simulink model "MPC"  (R2024b)
settings: Solver=ode4  StartTime=0.0  StopTime=tsim  FixedStep=baseRate  RelTol=1e-6  AbsTol=1e-6
values from neighbouring files (symbols this model uses):
  C = [cos(theta), -sin(theta) ... (first row only)    [Run_Initializer.m]    (also in plotBatch.m = quat2Rotm(q','scalarFirst'))
  camera_FOV = 40*d2r    (= 0.698131700798)    [Run_Initializer.m]
  camera_offset = [0.145, 0.087]'    [Run_Initializer.m]
  docking_face = [0 1]'    [Run_Initializer.m]
  docking_offset = [0 0 0]'    [Run_Initializer.m]
  eta = 0.7    [Run_Initializer.m]
  F_t = [kron(eye(N_h),  [zeros(2,3), eye(2), zeros(2,4)]) ... (first row only)    [Run_Initializer.m]
  f_t = [kron(ones(N_h, 1), [xLength yLength]' - edge_buffer) ... (first row only)    [Run_Initializer.m]
  F_u = [kron(eye(N_h),  [eye(3), zeros(3,6)]) ... (first row only)    [Run_Initializer.m]
  f_u = kron(ones(2*N_h, 1), u_max')    [Run_Initializer.m]
  F_v = [kron(eye(N_h),  [zeros(1,5), 1, zeros(1,3)]) ... (first row only)    [Run_Initializer.m]
  gamma = 0.95    [Run_Initializer.m]
  Gamma1_el = 0.12    [Run_Initializer.m]
  Gamma1_sh = 0.005    [Run_Initializer.m]
  Gamma1_wr = 0.025    [Run_Initializer.m]
  Gamma2_el = 5    [Run_Initializer.m]
  Gamma2_sh = 5    [Run_Initializer.m]
  Gamma2_wr = 5    [Run_Initializer.m]
  Gamma3_el = 10    [Run_Initializer.m]
  Gamma3_sh = 40    [Run_Initializer.m]
  Gamma3_wr = 40    [Run_Initializer.m]
  Gamma4_el = 0.039    [Run_Initializer.m]
  Gamma4_sh = 0.015    [Run_Initializer.m]
  Gamma4_wr = 0.029    [Run_Initializer.m]
  Gamma5_el = 800    [Run_Initializer.m]
  Gamma5_sh = 800    [Run_Initializer.m]
  Gamma5_wr = 800    [Run_Initializer.m]
  Gamma6_el = 0.000001    (= 1e-06)    [Run_Initializer.m]
  Gamma6_sh = 0.005    [Run_Initializer.m]
  Gamma6_wr = 0.02    [Run_Initializer.m]
  H = kron(eye(N_h), [R, zeros(3,6); zeros(6,3), Q])    [Run_Initializer.m]
  IBLACK = 0.1996    [unpackData.m]
  IRED = 0.1982    [unpackData.m]
  J = sum(wp*posErr + wt*angErr)    [find_transformation.m]
  Kd_elarm = 0.8    [Run_Initializer.m]
  Kd_sharm = 1.0    (= 1)    [Run_Initializer.m]
  Kd_wrarm = 0.6    [Run_Initializer.m]
  Kp_elarm = 1.2    [Run_Initializer.m]
  Kp_sharm = 1.5    [Run_Initializer.m]
  Kp_wrarm = 1.0    (= 1)    [Run_Initializer.m]
  m = m + 5    (= 4)    [unpackData.m]
  M = diag([1/m; 1/m; 1/I])    [unpackData.m]
  maxd = [d1 ... (first row only)    [Run_Initializer.m]
  mBLACK = 11.3620    (= 11.362)    [unpackData.m]
  mRED = 11.2970    (= 11.297)    [unpackData.m]
  N = size(rel,1)    [plotBatch.m]    (also in unpackData.m = 0)
  p = [0 obj.pos(k,:)]    [SparseState6DOF.m]
  PDQ = blkdiag(20*eye(3),eye(3), 20*eye(3),eye(3))    [Run_Initializer.m]
  PQ = blkdiag(20*eye(6),eye(6))    [Run_Initializer.m]
  PR = blkdiag(20*eye(3), eye(6), 0.0001*eye(3))    [Run_Initializer.m]
  PWMFreq = 5    [Run_Initializer.m]
  Q = diag([100 100 100 300 300 300])    [Run_Initializer.m]    (also in unpackData.m = blkdiag(0.0001*eye(2), 0.00001))
  R = diag([200 200 200])    [Run_Initializer.m]    (also in plotBatch.m = C3(yaw); unpackData.m = diag([6;6;6]))
  r_hold_obs = 1.1*sqrt(2)*0.3.*[1 1]    [Run_Initializer.m]
  r_hold_tar_min = [0.8; (0.3+0.05)]    [Run_Initializer.m]
  rho = 0.98    [Run_Initializer.m]
  T_d = 2    [Run_Initializer.m]
  T_max = 0.15    [Run_Initializer.m]
  Tz_lim_elarm = .1    (= 0.1)    [Run_Initializer.m]
  Tz_lim_sharm = .1    (= 0.1)    [Run_Initializer.m]
  Tz_lim_wrarm = .1    (= 0.1)    [Run_Initializer.m]
  use_LOS_constr = 1    [Run_Initializer.m]
  use_table_constr = 1    [Run_Initializer.m]
  x_BLACK_0 = [(1/3)*xLength (1/3)*yLength-0.2 280*d2r 0.01 0.005 1.88*d2r]'    [Run_Initializer.m]
  x_BLUE_0 = [0 0 0 0 0 0]'    [Run_Initializer.m]
  zeta = 10*d2r    (= 0.174532925199)    [Run_Initializer.m]
undefined symbols (not defined in the file or in its folder): a1, a2, a3, alpha, alpha_m, alpha_t, alphas, alphas_t, alphat, Am, b, b0, b1, b2, b3, baseRate, Bm, c, c1, c1t, c2, c2t, Cm, d, dataRate, DiscIntNeverNeededParam, Dm, drop_states_ARM, drop_states_BLACK, drop_states_BLUE, drop_states_RED, epsilon, epsilont, F_black_X_nominal, F_black_Y_nominal, F_blue_X_nominal, F_blue_Y_nominal, F_max, F_red_X_nominal, F_red_Y_nominal, F_thrusters_BLACK, F_thrusters_BLUE, F_thrusters_RED, gamma_I, gamma_I_t, gamma_P, gamma_P_t, home_states_BLACK, home_states_BLUE, home_states_RED, IBLUE, IDIST, IEE, init_states_BLACK, init_states_BLUE, init_states_RED, IPROX, k, K, k1 ... (+62)
libraries: simulink x33, nvidiaSharedBlocks x13, slpidlib x6, MainLibrary x5, dspsigops x3, dspinverses x3, nvidiaIMUSensorslib x1
(part 10 of 12)

== system MPC/Thruster Control Code/Change RED Behavior/Calculate Duty Cycle/Duty Cycle @ PWM/Enabled Subsystem1 ==
  ThrustPer_Final : Inport
  Enable : EnablePort
  Out1 : Outport
  wires:
  ThrustPer_Final/1 -> Out1/1

== system MPC/1 - Experiment Logic/Phase #3: Experiment/Sub-Phase #1/Desired Position BLACK/Calculate Time since Phase #3 Start/Subsystem ==
  Universal_Time : DataStoreRead  DataStoreName=Univ_Time  IndexOptions=Index vector (dialog)  Indices=1  OutputSizes=1
  Time : Outport  VectorParamsAs1DForOutWhenUnconnected=off
  wires:
  Universal_Time/1 -> Time/1

== system MPC/1 - Experiment Logic/Phase #3: Experiment/Sub-Phase #1/Desired Position BLUE/Calculate Time since Phase #3 Start/Subsystem ==
  Universal_Time : DataStoreRead  DataStoreName=Univ_Time  IndexOptions=Index vector (dialog)  Indices=1  OutputSizes=1
  Time : Outport  VectorParamsAs1DForOutWhenUnconnected=off
  wires:
  Universal_Time/1 -> Time/1

== system MPC/1 - Experiment Logic/Phase #3: Experiment/Sub-Phase #3 /Desired Position BLACK/Calculate Time since Phase #3 Start/Subsystem ==
  Universal_Time : DataStoreRead  DataStoreName=Univ_Time  IndexOptions=Index vector (dialog)  Indices=1  OutputSizes=1
  Time : Outport  VectorParamsAs1DForOutWhenUnconnected=off
  wires:
  Universal_Time/1 -> Time/1

== system MPC/1 - Experiment Logic/Phase #3: Experiment/Sub-Phase #4/Desired Position BLACK/Calculate Time since Phase #3 Start/Subsystem ==
  Universal_Time : DataStoreRead  DataStoreName=Univ_Time  IndexOptions=Index vector (dialog)  Indices=1  OutputSizes=1
  Time : Outport  VectorParamsAs1DForOutWhenUnconnected=off
  wires:
  Universal_Time/1 -> Time/1

== system MPC/4 - Control/Default PD Control (RED)/SAC/SAC_CTL/Position/Storage ==
  u : Inport
  In2 : Inport  Port=2
  u1 : Inport  Port=3
  Data Store Write : DataStoreWrite  DataStoreName=SAC_ke_1  IndexOptions=Index vector (dialog)  Indices=1  OutputSizes=1
  Data Store Write1 : DataStoreWrite  DataStoreName=SAC_kx_1  IndexOptions=Index vector (dialog)  Indices=1  OutputSizes=1
  Data Store Write10 : DataStoreWrite  DataStoreName=SAC_kx_3  IndexOptions=Index vector (dialog)  Indices=1  OutputSizes=1
  Data Store Write11 : DataStoreWrite  DataStoreName=SAC_kx_4  IndexOptions=Index vector (dialog)  Indices=1  OutputSizes=1
  Data Store Write12 : DataStoreWrite  DataStoreName=SAC_kx_5  IndexOptions=Index vector (dialog)  Indices=1  OutputSizes=1
  Data Store Write13 : DataStoreWrite  DataStoreName=SAC_kx_6  IndexOptions=Index vector (dialog)  Indices=1  OutputSizes=1
  Data Store Write14 : DataStoreWrite  DataStoreName=SAC_kx_7  IndexOptions=Index vector (dialog)  Indices=1  OutputSizes=1
  Data Store Write15 : DataStoreWrite  DataStoreName=SAC_kx_8  IndexOptions=Index vector (dialog)  Indices=1  OutputSizes=1
  Data Store Write2 : DataStoreWrite  DataStoreName=SAC_ku_1  IndexOptions=Index vector (dialog)  Indices=1  OutputSizes=1
  Data Store Write3 : DataStoreWrite  DataStoreName=SAC_ke_2  IndexOptions=Index vector (dialog)  Indices=1  OutputSizes=1
  Data Store Write4 : DataStoreWrite  DataStoreName=SAC_ke_3  IndexOptions=Index vector (dialog)  Indices=1  OutputSizes=1
  Data Store Write5 : DataStoreWrite  DataStoreName=SAC_ke_4  IndexOptions=Index vector (dialog)  Indices=1  OutputSizes=1
  Data Store Write6 : DataStoreWrite  DataStoreName=SAC_ku_2  IndexOptions=Index vector (dialog)  Indices=1  OutputSizes=1
  Data Store Write7 : DataStoreWrite  DataStoreName=SAC_ku_3  IndexOptions=Index vector (dialog)  Indices=1  OutputSizes=1
  Data Store Write8 : DataStoreWrite  DataStoreName=SAC_ku_4  IndexOptions=Index vector (dialog)  Indices=1  OutputSizes=1
  Data Store Write9 : DataStoreWrite  DataStoreName=SAC_kx_2  IndexOptions=Index vector (dialog)  Indices=1  OutputSizes=1
  MATLAB Function : MATLAB Function  TreatAsAtomicUnit=on
  MATLAB Function1 : MATLAB Function  TreatAsAtomicUnit=on
  MATLAB Function2 : MATLAB Function  TreatAsAtomicUnit=on
  MATLAB Function3 : MATLAB Function  TreatAsAtomicUnit=on
  MATLAB Function4 : MATLAB Function  TreatAsAtomicUnit=on
  wires:
  MATLAB Function2/3(y3) -> Data Store Write7/1
  u1/1 -> MATLAB Function2/1(u)
  MATLAB Function/3(y3) -> Data Store Write4/1
  MATLAB Function2/4(y4) -> Data Store Write8/1
  MATLAB Function2/1(y1) -> Data Store Write2/1
  MATLAB Function/4(y4) -> Data Store Write5/1
  MATLAB Function/1(y1) -> Data Store Write/1
  MATLAB Function/2(y2) -> Data Store Write3/1
  MATLAB Function2/2(y2) -> Data Store Write6/1
  u/1 -> MATLAB Function/1(u)
  MATLAB Function3/1(y1) -> Data Store Write1/1
  In2/1 -> MATLAB Function4/1(u)
  MATLAB Function4/1(y1) -> MATLAB Function3/1(u)
  MATLAB Function4/2(y2) -> MATLAB Function1/1(u)
  MATLAB Function3/2(y2) -> Data Store Write9/1
  MATLAB Function3/3(y3) -> Data Store Write10/1
  MATLAB Function1/1(y1) -> Data Store Write12/1
  MATLAB Function3/4(y4) -> Data Store Write11/1
  MATLAB Function1/2(y2) -> Data Store Write13/1
  MATLAB Function1/3(y3) -> Data Store Write14/1
  MATLAB Function1/4(y4) -> Data Store Write15/1

== system MPC/Simulate Plant Dynamics/RED and ARM Dynamics/RED + ARM/Calculated & Store Measured States/Subsystem3/Enabled Subsystem ==
  y : Inport
  dt : Inport  Port=2
  Enable : EnablePort
  Constant2 : Constant  Value=0.1
  Delay : Delay  DelayLength=1  InitialConditionSource=Input port
      settings: InputPortMap=u0,p4
  Delay1 : Delay  DelayLength=1
  MATLAB Function : MATLAB Function  TreatAsAtomicUnit=on
  dy/dt : Outport
  wires:
  Constant2/1 -> MATLAB Function/3(tau)
  dt/1 -> MATLAB Function/2(dt)
  Delay/1 -> MATLAB Function/5(ema_prev)
  Delay1/1 -> MATLAB Function/4(dy_prev)
  MATLAB Function/2(ema) -> Delay/1
  y/1 -> MATLAB Function/1(y), Delay/2
  MATLAB Function/1(dy) -> Delay1/1, dy/dt/1

== system MPC/Simulate Plant Dynamics/RED and ARM Dynamics/RED + ARM/Calculated & Store Measured States/Subsystem4/Enabled Subsystem ==
  y : Inport
  dt : Inport  Port=2
  Enable : EnablePort
  Constant2 : Constant  Value=0.1
  Delay : Delay  DelayLength=1  InitialConditionSource=Input port
      settings: InputPortMap=u0,p4
  Delay1 : Delay  DelayLength=1
  MATLAB Function : MATLAB Function  TreatAsAtomicUnit=on
  dy/dt : Outport
  wires:
  Constant2/1 -> MATLAB Function/3(tau)
  dt/1 -> MATLAB Function/2(dt)
  Delay/1 -> MATLAB Function/5(ema_prev)
  Delay1/1 -> MATLAB Function/4(dy_prev)
  MATLAB Function/2(ema) -> Delay/1
  y/1 -> MATLAB Function/1(y), Delay/2
  MATLAB Function/1(dy) -> Delay1/1, dy/dt/1

== system MPC/Simulate Plant Dynamics/RED and ARM Dynamics/RED + ARM/Calculated & Store Measured States/Subsystem5/Enabled Subsystem ==
  y : Inport
  dt : Inport  Port=2
  Enable : EnablePort
  Constant2 : Constant  Value=0.1
  Delay : Delay  DelayLength=1  InitialConditionSource=Input port
      settings: InputPortMap=u0,p4
  Delay1 : Delay  DelayLength=1
  MATLAB Function : MATLAB Function  TreatAsAtomicUnit=on
  dy/dt : Outport
  wires:
  Constant2/1 -> MATLAB Function/3(tau)
  dt/1 -> MATLAB Function/2(dt)
  Delay/1 -> MATLAB Function/5(ema_prev)
  Delay1/1 -> MATLAB Function/4(dy_prev)
  MATLAB Function/2(ema) -> Delay/1
  y/1 -> MATLAB Function/1(y), Delay/2
  MATLAB Function/1(dy) -> Delay1/1, dy/dt/1

== system MPC/Simulate Plant Dynamics/RED and ARM Dynamics/RED + ARM/Data @ Measurement Rate/Calculate True Time Step/Enabled Subsystem3 ==
  y2-y1 : Inport
  Enable : EnablePort
  dy(t)/dt : Outport
  wires:
  y2-y1/1 -> dy(t)/dt/1

== system MPC/Simulate Plant Dynamics/RED and ARM Dynamics/RED Only/Calculated & Store Measured States/Subsystem1/Enabled Subsystem ==
  y : Inport
  dt : Inport  Port=2
  Enable : EnablePort
  Constant2 : Constant  Value=0.1
  Delay : Delay  DelayLength=1  InitialConditionSource=Input port
      settings: InputPortMap=u0,p4
  Delay1 : Delay  DelayLength=1
  MATLAB Function : MATLAB Function  TreatAsAtomicUnit=on
  dy/dt : Outport
  wires:
  Constant2/1 -> MATLAB Function/3(tau)
  dt/1 -> MATLAB Function/2(dt)
  Delay/1 -> MATLAB Function/5(ema_prev)
  Delay1/1 -> MATLAB Function/4(dy_prev)
  MATLAB Function/2(ema) -> Delay/1
  y/1 -> MATLAB Function/1(y), Delay/2
  MATLAB Function/1(dy) -> Delay1/1, dy/dt/1

== system MPC/Simulate Plant Dynamics/RED and ARM Dynamics/RED Only/Calculated & Store Measured States/Subsystem2/Enabled Subsystem ==
  y : Inport
  dt : Inport  Port=2
  Enable : EnablePort
  Constant2 : Constant  Value=0.1
  Delay : Delay  DelayLength=1  InitialConditionSource=Input port
      settings: InputPortMap=u0,p4
  Delay1 : Delay  DelayLength=1
  MATLAB Function : MATLAB Function  TreatAsAtomicUnit=on
  dy/dt : Outport
  wires:
  Constant2/1 -> MATLAB Function/3(tau)
  dt/1 -> MATLAB Function/2(dt)
  Delay/1 -> MATLAB Function/5(ema_prev)
  Delay1/1 -> MATLAB Function/4(dy_prev)
  MATLAB Function/2(ema) -> Delay/1
  y/1 -> MATLAB Function/1(y), Delay/2
  MATLAB Function/1(dy) -> Delay1/1, dy/dt/1

== system MPC/Simulate Plant Dynamics/RED and ARM Dynamics/RED Only/Data @ Measurement Rate/Calculate True Time Step/Enabled Subsystem3 ==
  y2-y1 : Inport
  Enable : EnablePort
  dy(t)/dt : Outport
  wires:
  y2-y1/1 -> dy(t)/dt/1

== matlab function MPC/Data Logger Subsystem/Subsystem8/MATLAB Function ==
  data: u input; y output
function y = fcn(u)

if anynan(u)
    y = -1*ones(size(u));
else
    y = u;
end
end

== matlab function MPC/3 - Navigation/Subsystem/STQMEKF1/MATLAB Function2 ==
  data: u input; out output
function out = fcn(u)

y = u;

y(1:4) = smallQuat(u(1:4),'scalarFirst');
y(5:7) = -1*u(5:7);

out = [y(1:4); y(8:10); y(5:7); y(11:13)];

== matlab function MPC/3 - Navigation/Subsystem/STRMEKF1/MATLAB Function ==
  data: x input; out output; q input
function out = fcn(x,q)

y = [q;x];
y(1:4) = smallQuat(y(1:4),'scalarFirst');

out = [y(1:7); y(11:13); y(8:10)];

== matlab function MPC/Data Logger Subsystem/Subsystem17/MATLAB Function ==
  data: u input; y output
function y = fcn(u)

if anynan(u)
    y = -1*ones(size(u));
else
    y = u;
end
end

== matlab function MPC/Data Logger Subsystem/Subsystem11/MATLAB Function ==
  data: u input; y output
function y = fcn(u)

if anynan(u)
    y = -1*ones(size(u));
else
    y = u;
end
end

== matlab function MPC/3 - Navigation/Subsystem/STRMEKF1/MATLAB Function1 ==
  data: dt input; RED_yaw input; RED_x input; VIS_R input; VIS_x input; x_est output; Rot_est output; x_prev input; Rot_prev input; P_prev input; P_est output; compT output; y output; NIS output; V_est output; V_prev input; Q parameter; R parameter; maxd parameter
function [x_est, Rot_est, P_est, compT, y, NIS, V_est] = RMEKF(dt, RED_yaw, RED_x, VIS_R, VIS_x, x_prev, Rot_prev, P_prev, V_prev, Q, R, maxd)

s1 = 1e-2; % quat
s2 = 1e-4; % angular vel
s3 = 1e-10; % position
s4 = 1e-7; % velocity
s5 = 0.006; % quat meas 
s6 = 0.001 ; % position meas
s7 = s6; 

d1 = 1.6046;
d2 = 5.5866;
rho = 0.98;

Q = blkdiag(s1*eye(3), s3*eye(3), s4*eye(3), s2*eye(3));


R = blkdiag(s5*eye(3), s6, s7*eye(2));

maxd = 1000*[d1
        d2];

rho = 0.98;

r = 0;
z = VIS_x;
Chaser = [RED_x(1:2); RED_yaw];

tic
[x_est, Rot_est, P_est, y, H, V_est] = runSTRMEKF2(Chaser, z, VIS_R, dt, x_prev, Rot_prev, P_prev, Q, R, V_prev, r, rho, maxd);

compT = toc;

% Calc NIS
Pzz = H*P_est*H' + R;
NIS = y' / Pzz * y;

end

== matlab function MPC/Data Logger Subsystem/Subsystem13/MATLAB Function ==
  data: u input; y output
function y = fcn(u)

if anynan(u)
    y = -1*ones(size(u));
else
    y = u;
end
end

== matlab function MPC/Data Logger Subsystem/Subsystem14/MATLAB Function ==
  data: u input; y output
function y = fcn(u)

if anynan(u)
    y = -1*ones(size(u));
else
    y = u;
end
end

== matlab function MPC/3 - Navigation/Subsystem/STRMEKF1/MATLAB Function11 ==
  data: u input; y output
function y = fcn(u)
if det(u) == 0
    u = eye(3);
end
u(1:2,1:2) = u(1:2,1:2);
y = rotm2Quat(u','scalarFirst');

== matlab function MPC/Data Logger Subsystem/Subsystem2/MATLAB Function ==
  data: u input; y output
function y = fcn(u)

if anynan(u)
    y = -1*ones(size(u));
else
    y = u;
end
end

== matlab function MPC/Data Logger Subsystem/Subsystem5/MATLAB Function ==
  data: u input; y output
function y = fcn(u)

if anynan(u)
    y = -1*ones(size(u));
else
    y = u;
end
end

== matlab function MPC/Data Logger Subsystem/Subsystem6/MATLAB Function ==
  data: u input; y output
function y = fcn(u)

if anynan(u)
    y = -1*ones(size(u));
else
    y = u;
end
end

== matlab function MPC/Receive Data /Subsystem/MATLAB Function ==
  data: u input; p_cam output
function p_cam = fcn(u)
tx = 0.3825;
ty = -0.0378;
theta_cam = 0.1483 - 0.075;

R_cam = [cos(theta_cam), -sin(theta_cam), 0; sin(theta_cam), cos(theta_cam), 0; 0, 0, 1];
t_cam = [tx; ty; 0];

p_cam = R_cam * u + t_cam;

== matlab function MPC/Receive Data /Subsystem/MATLAB Function3 ==
  data: u input; y output
function y = fcn(u)
theta_cam = 0.1483 - 0.075;

y = wrapToPi(-theta_cam/2 + u);

== matlab function MPC/Receive Data /Subsystem/MATLAB Function4 ==
  data: z input; x output; zk input
function x = fcn(z,zk)

if sum(abs(z - zk)) < 10^-10
    x = NaN(size(z));
else
    x = z;
end
end

== matlab function MPC/Receive Data /Subsystem/MATLAB Function5 ==
  data: u input; y output
function y = fcn(u)
theta_cam = 0.1483 - 0.075;

y = wrapToPi(-theta_cam/2 + u);

== matlab function MPC/PhaseSpace Filter Code/Subsystem2/Subsystem/MATLAB Function1 ==
  data: u input; y output; uprev input
function y = fcn(u, uprev)
    if sum(abs(u-uprev)) < 10^-10
        y = NaN(3,1);
    else
        y = [u(1:2);unwrap(u(3))];
    end
end

== matlab function MPC/Receive Data /Subsystem/MATLAB Function6 ==
  data: u input; p_cam output
function p_cam = fcn(u)
tx = 0.3825;
ty = -0.0378;
theta_cam = 0.1483 - 0.075;

R_cam = [cos(theta_cam), -sin(theta_cam), 0; sin(theta_cam), cos(theta_cam), 0; 0, 0, 1];
t_cam = [tx; ty; 0];

p_cam = R_cam * u + t_cam;

== matlab function MPC/Receive Data /Subsystem/MATLAB Function1 ==
  data: z input; x output; zk input
function x = fcn(z,zk)

if sum(abs(z - zk)) < 10^-10
    x = NaN(size(z));
else
    x = z;
end
end

== matlab function MPC/Receive Data /Subsystem/MATLAB Function2 ==
  data: z input; x output; zk input
function x = fcn(z,zk)

if sum(abs(z - zk)) < 10^-10
    x = NaN(size(z));
else
    x = z;
end
end

== matlab function MPC/Receive Data /Subsystem/Pose2/MATLAB Function ==
  data: x input; yaw input; dq output; q output; R output
function [dq,q,R] = fcn(x,yaw)
    R = C3(yaw);
    T = [R, x; zeros(1,3), 1];
    q = rotm2Quat(R,'scalarFirst');
    dq = htform2Dq(T,'scalarFirst');
end

== matlab function MPC/Receive Data /Subsystem/Pose1/MATLAB Function ==
  data: x input; yaw input; dq output; q output; R output
function [dq,q,R] = fcn(x, yaw)
    R = C3(yaw);
    T = [R, x; zeros(1,3), 1];
    T = htformInverse(T);
    
    q = rotm2Quat(R,'scalarFirst');
    dq = htform2Dq(T,'scalarFirst');
end

== matlab function MPC/3 - Navigation/Subsystem/MATLAB Function11 ==
  data: q_red input; q_vis input; y output; v input; x input
function y = fcn(q_red, q_vis, v, x)

if isfinite(q_vis)
    q_black = quatMultiply(q_vis,q_red,'scalarFirst');
    q_black = smallQuat(q_black,'scalarFirst');
else
    q_black = NaN(4,1);
end

v = quatRotate(q_red,v,'scalarFirst');
temp = v + x;

y = [q_black; temp];

== matlab function MPC/3 - Navigation/Subsystem/MATLAB Function12 ==
  data: q_red input; q_vis input; y output; v input; x input
function y = fcn(q_red, q_vis, v, x)

if isfinite(q_vis)
    q_black = quatMultiply(q_vis,q_red,'scalarFirst');
    q_black = smallQuat(q_black,'scalarFirst');
else
    q_black = NaN(4,1);
end

v = quatRotate(q_red,v,'scalarFirst');
temp = v + x;

y = [q_black; temp];

== matlab function MPC/3 - Navigation/Subsystem/DQMEKF/MATLAB Function1 ==
  data: dt input; RED_dq input; VIS_dq input; x_est output; x_prev input; P_prev input; P_est output; compT output; Q parameter; R parameter; maxd parameter; y output; NIS output
function [x_est, P_est, compT, y, NIS] = DQMEKF(dt, RED_dq, VIS_dq, x_prev, P_prev, Q, R, maxd)

s1 = 1e-6;
s2 = 1e-6;
s3 = 1e-10;
s4 = 1e-7 ;
s5 = 0.06;
s6 = 0.001 ;
s7 = s6;

d1 = 1.6046;
d2 = 5.5866;

Q = blkdiag(s1*eye(3), s3*eye(3), s2*eye(3), s4*eye(3));


R = blkdiag(s5*eye(3), s6, s7*eye(2));

maxd = [d1
        d2];
r = 0;
z = VIS_dq;
Chaser = RED_dq;

tic
[x_est, P_est, y, H] = runDQMEKF(z, dt, ...
       x_prev, P_prev, Q, R, r, maxd, Chaser);
compT = toc;

Pzz = H*P_est*H' + R;
NIS = y' / Pzz * y;
end

== matlab function MPC/4 - Control/Default LQR Control (BLUE)/Calculate Error/MATLAB Function ==
  data: Rz_path input; Rz_error output; Rz_measured input
function Rz_error = SmoothAngularDifference(Rz_path, Rz_measured)

    Rz_error = mod(Rz_measured-Rz_path+pi, 2*pi)-pi;


end

== matlab function MPC/3 - Navigation/Subsystem/DQMEKF/MATLAB Function3 ==
  data: u input; x output
function x = fcn(u)
dq = [u(1:4),u(5:8)];
dv = [[0; u(9:11)], [0; u(12:14)]];
if norm(dq(:,1)) == 0
    dq = zeros(4,2);
    dq(1,1) = 1;
end
[q,r] = dq2quat(dq,'scalarFirst');
q = smallQuat(q,'scalarFirst');
v = dqLinearVelocity(dv, dq);
w = dv(2:4,1);
x = [q; r'; -w; -v];
end

function v_world = dqLinearVelocity(dq_vel, dq_pose)


    %-- 1) body‐frame linear velocity (pure quaternion) --%
    % Conjugate of the pose rotation quaternion:
    q_r_conj = quatConj(dq_pose(:,1),'scalarFirst');
    
    % pure‐quat v_body_q = 2 * (qv_dual * conj(q_pose.r))
    v_body_quat = 2 * quatMultiply(dq_vel(:,2), q_r_conj,'scalarFirst');
    
    %-- 2) rotate into world frame --%
    % dqRotate(q, p) ≡ q * p * conj(q) v_body_quat(2:4)
    v_world_quat = quatRotate(dq_pose(:,1), v_body_quat(2:4),'scalarFirst');
    
    %-- 3) extract vector part --%
    v_world = v_world_quat;

end

== matlab function MPC/4 - Control/Default PD Control (RED)/CSMC/MATLAB Function4 ==
  data: q2 input; u output; k1 parameter; alpha parameter
function u = fcn(q2,k1, alpha)

u = sign(k1*q2)*(abs(k1*q2)^alpha);

== matlab function MPC/4 - Control/Default PD Control (RED)/CSMC/MATLAB Function5 ==
  data: q1 input; phi output; k1 parameter; alpha parameter; q2 input
function phi = fcn(q1,k1, alpha, q2)



phi = k1*q1 + (1/(2 - alpha))*sign(k1*q2)*(abs(k1*q2))^(2 - alpha);

== matlab function MPC/4 - Control/Default PD Control (RED)/CSMC/MATLAB Function6 ==
  data: phi input; u output; alpha parameter
function u = fcn(phi, alpha)



u = sign(phi)*(abs(phi)^(alpha/(2 - alpha)));

== matlab function MPC/PhaseSpace Camera Code/Use Hardware to Obtain States/Receive and Process Phasespace Data/Check for Sychronization/MATLAB Function ==
  data: StartClock output; RedReceiving input; BlackReceiving input; BlueReceiving input; platformSelection parameter
function StartClock = CheckForSync(RedReceiving, BlackReceiving, BlueReceiving, platformSelection)
        
    StartClock = 0;
    
    if (platformSelection == 1)
        
        if RedReceiving == 1

            StartClock = 1;

        else

            StartClock = 0;

        end
        
    elseif (platformSelection == 2)
        
        if BlackReceiving == 1

            StartClock = 1;

        else

            StartClock = 0;

        end  
        
    elseif (platformSelection == 3)
        
        if RedReceiving == 1 && BlackReceiving == 1

            StartClock = 1;

        else

            StartClock = 0;

        end    
        
    elseif (platformSelection == 4)
        
        if RedReceiving == 1 && BlackReceiving == 1

            StartClock = 1;

        else

            StartClock = 0;

        end
        
    elseif (platformSelection == 5)
        
        if RedReceiving == 1

            StartClock = 1;

        else

            StartClock = 0;

        end
        
    elseif (platformSelection == 6)
        
        if BlueReceiving == 1

            StartClock = 1;

        else

            StartClock = 0;

        end
        
    elseif (platformSelection == 7)
        
        if RedReceiving == 1 && BlueReceiving == 1

            StartClock = 1;

        else

            StartClock = 0;

        end
        
    elseif (platformSelection == 8)
        
        if RedReceiving == 1 && BlackReceiving == 1 && BlueReceiving == 1

            StartClock = 1;

        else

            StartClock = 0;

        end
        
    elseif (platformSelection == 9)
        
        if BlackReceiving == 1 && BlueReceiving == 1

            StartClock = 1;

        else

            StartClock = 0;

        end
                           
    elseif (platformSelection == 10)
        
        if RedReceiving == 1 && BlueReceiving == 1

            StartClock = 1;

        else

            StartClock = 0;

        end
        
    elseif (platformSelection == 11)
        
        if RedReceiving == 1 && BlackReceiving == 1 && BlueReceiving == 1

            StartClock = 1;

        else

            StartClock = 0;

        end
        
    end



end

== matlab function MPC/4 - Control/Default PD Control (RED)/CSMC/MATLAB Function7 ==
  data: q2 input; u output; k1 parameter; alpha parameter
function u = fcn(q2,k1, alpha)

u = sign(k1*q2)*(abs(k1*q2)^alpha);

== matlab function MPC/4 - Control/Default PD Control (RED)/CSMC/MATLAB Function8 ==
  data: q1 input; phi output; k1 parameter; alpha parameter; q2 input
function phi = fcn(q1,k1, alpha, q2)



phi = k1*q1 + (1/(2 - alpha))*sign(k1*q2)*(abs(k1*q2))^(2 - alpha);

== matlab function MPC/4 - Control/Default PD Control (RED)/DAC Controller/Fx Gain Derivatives ==
  data: e_xdot input; k2_dot output; e_x input; k1_dot output; lambda1 parameter; lambda2 parameter; lambda12 parameter; p parameter
function [k2_dot, k1_dot]= fcn(e_xdot, e_x, lambda1, lambda2, lambda12, p)

k1_dot = -lambda1*p*e_x^2-(lambda1+p*lambda12)*e_x*e_xdot-lambda12*e_xdot^2;
k2_dot = -lambda12*p*e_x^2-(lambda12+p*lambda2)*e_x*e_xdot-lambda2*e_xdot^2;

== matlab function MPC/4 - Control/Default PD Control (BLUE)/Calculate Error/MATLAB Function ==
  data: Rz_path input; Rz_error output; Rz_measured input
function Rz_error = SmoothAngularDifference(Rz_path, Rz_measured)

    Rz_error = mod(Rz_measured-Rz_path+pi, 2*pi)-pi;


end

== matlab function MPC/3 - Navigation/Subsystem/QMEKF/MATLAB Function ==
  data: u input; out output
function out = fcn(u)

y = u;

y(1:4) = smallQuat(u(1:4),'scalarFirst');
y(5:7) = -1*u(5:7);

out = [y(1:4); y(8:10); y(5:7); y(11:13)];

== matlab function MPC/4 - Control/Default PD Control (RED)/DAC Controller/Fy Gain Derivatives ==
  data: k2_dot output; e_ydot input; e_y input; k1_dot output; lambda1 parameter; lambda2 parameter; lambda12 parameter; p parameter
function [k2_dot, k1_dot]= fcn(e_ydot, e_y, lambda1, lambda2, lambda12, p)

k1_dot = -lambda1*p*e_y^2-(lambda1+p*lambda12)*e_y*e_ydot-lambda12*e_ydot^2;
k2_dot = -lambda12*p*e_y^2-(lambda12+p*lambda2)*e_y*e_ydot-lambda2*e_ydot^2;

== matlab function MPC/4 - Control/Default PD Control (RED)/DAC Controller/Torque Gain Derivatives ==
  data: e_t input; e_tdot input; k1_dot output size=1; k2_dot output size=1; lambda1_t parameter; lambda2_t parameter; lambda12_t parameter; p_t parameter
function [k1_dot, k2_dot]= fcn(e_t, e_tdot, lambda1_t, lambda2_t, lambda12_t, p_t)
k1_dot = -lambda1_t*p_t*e_t^2-(lambda1_t+p_t*lambda12_t)*e_t*e_tdot-lambda12_t*e_tdot^2;
k2_dot = -lambda12_t*p_t*e_t^2-(lambda12_t+p_t*lambda2_t)*e_t*e_tdot-lambda2_t*e_tdot^2;

== matlab function MPC/4 - Control/Default PD Control (RED)/Homo/MATLAB Function ==
  data: q1 input; u output; k1 parameter; alpha parameter
function u = fcn(q1,k1, alpha)

u = k1*sign(q1)*(abs(q1)^(alpha/(2 - alpha)));

== matlab function MPC/4 - Control/Default PD Control (RED)/Homo/MATLAB Function1 ==
  data: q2 input; u output; k2 parameter; alpha parameter
function u = fcn(q2,k2, alpha)

u = k2*sign(q2)*(abs(q2)^alpha);

== matlab function MPC/4 - Control/Default PD Control (RED)/Homo/MATLAB Function2 ==
  data: q1 input; u output; k1 parameter; alpha parameter
function u = fcn(q1,k1, alpha)

u = k1*sign(q1)*(abs(q1)^(alpha/(2 - alpha)));

== matlab function MPC/3 - Navigation/Subsystem/QMEKF/MATLAB Function1 ==
  data: dt input; RED_quat input; RED_x input; BLACK_q input; BLACK_x input; x_est output; x_prev input; P_prev input; P_est output; compT output; y output; NIS output; Q parameter; R parameter; maxd parameter
function [x_est, P_est,compT,y,NIS] = QMEKF(dt, RED_quat, RED_x, BLACK_q, BLACK_x, x_prev, P_prev, Q, R, maxd)

%% Best QMEKF values
s1 = 1e-6;
s2 = 1e-6;
s3 = 1e-10;
s4 = 1e-7 ;
s5 = 0.06;
s6 = 0.001 ;
s7 = s6;

d1 = 1.6046;
d2 = 5.5866;

Q = blkdiag(s1*eye(3), s2*eye(3), s3*eye(3), s4*eye(3));


R = blkdiag(s5*eye(3), s6, s7*eye(2));

maxd = [d1
        d2];

%%
r = 0;
z = [BLACK_q; BLACK_x];
Chaser = [RED_quat; RED_x];

tic
[y, H, x_est, P_est] = runQMEKF(z, dt, Chaser, ...
       x_prev, P_prev, Q, R, r, maxd);
compT = toc;


% Assume H is the full measurement matrix
H_att = H;  % Attitude submatrix
y_att = y;    % Attitude innovation
S_att = H_att * P_est * H_att' + R;
NIS = y_att' / S_att * y_att;


end

== matlab function MPC/Simulate Plant Dynamics/RED and ARM Dynamics/RED Only/Calculated & Store Measured States/Subsystem1/Enabled Subsystem/MATLAB Function ==
  data: y input; dy output; dt input; tau input; dy_prev input; ema_prev input; ema output
function [dy, ema] = realtime_derivative_ema(y, dt, tau, dy_prev, ema_prev)
    % Inputs:
    % y: Current measurement
    % dt: Time step
    % alpha: Smoothing factor (e.g., 0.1)

    alpha = 1 - exp(-dt / tau);
        
    % Update EMA
    ema = alpha.*y + (1 - alpha).*ema_prev;
    
    % Compute derivative
    dy = (ema - ema_prev)./dt;
    
end

== matlab function MPC/3 - Navigation/Subsystem/RMEKF/MATLAB Function ==
  data: x input; out output; q input
function out = fcn(x,q)

y = [q;x];
y(1:4) = smallQuat(y(1:4),'scalarFirst');

out = [y(1:7); y(11:13); y(8:10)];

== matlab function MPC/4 - Control/Default PD Control (RED)/Homo/MATLAB Function3 ==
  data: q2 input; u output; k2 parameter; alpha parameter
function u = fcn(q2,k2, alpha)

u = k2*sign(q2)*(abs(q2)^alpha);

== matlab function MPC/3 - Navigation/Subsystem/RMEKF/MATLAB Function1 ==
  data: dt input; RED_yaw input; RED_x input; VIS_R input; VIS_x input; x_est output; Rot_est output; x_prev input; Rot_prev input; P_prev input; P_est output; compT output; Q parameter; R parameter; maxd parameter; y output; NIS output
function [x_est, Rot_est, P_est,compT, y, NIS] = RMEKF(dt, RED_yaw, RED_x, VIS_R, VIS_x, x_prev, Rot_prev, P_prev, Q, R, maxd)

s1 = 1e-2; % quat
s2 = 1e-4; % angular vel
s3 = 1e-10; % position
s4 = 1e-7; % velocity
s5 = 0.006; % quat meas 
s6 = 0.001 ; % position meas
s7 = s6; 

d1 = 1.6046;
d2 = 5.5866;
rho = 0.98;

Q = blkdiag(s1*eye(3), s3*eye(3), s4*eye(3), s2*eye(3));


R = blkdiag(s5*eye(3), s6, s7*eye(2));

maxd = 1000*[d1
        d2];


r = 0;
z = VIS_x;
Chaser = [RED_x(1:2); RED_yaw];

tic
[x_est, Rot_est, P_est, y, H] = runRMEKF(Chaser, z, VIS_R, dt, x_prev, Rot_prev, P_prev, Q, R, r, maxd);
compT = toc;

% Calc Nis
Pzz = H*P_est*H' + R;
NIS = y' / Pzz * y;
end

== matlab function MPC/3 - Navigation/Subsystem/RMEKF/MATLAB Function11 ==
  data: u input; y output
function y = fcn(u)
if det(u) == 0
    u = eye(3);
end
u(1:2,1:2) = u(1:2,1:2);
y = rotm2Quat(u','scalarFirst');

== matlab function MPC/3 - Navigation/Subsystem/STDQMEKF/MATLAB Function1 ==
  data: dt input; RED_dq input; VIS_dq input; x_est output; x_prev input; P_prev input; P_est output; compT output; y output; NIS output; V_prev input; V_est output
function [x_est, P_est, compT, y, NIS, V_est] = STDQMEKF(dt, RED_dq, VIS_dq, x_prev, P_prev, V_prev)

s1 = 1e-6;
s2 = 1e-6;
s3 = 1e-10;
s4 = 1e-7 ;
s5 = 0.06;
s6 = 0.001 ;
s7 = s6;

d1 = 1.6046;
d2 = 5.5866;

Q = blkdiag(s1*eye(3), s3*eye(3), s2*eye(3), s4*eye(3));


R = blkdiag(s5*eye(3), s6, s7*eye(2));

rho = 0.98;

maxd = [d1
        d2];

r = 0;
z = VIS_dq;
Chaser = RED_dq;

tic
[x_est, P_est, y, H, V_est] = runSTDQMEKF(z, dt, ...
       x_prev, P_prev, Q, R, V_prev, r, rho, maxd, Chaser);
compT = toc;

Pzz = H*P_est*H' + R;
NIS = y' / Pzz * y;
end

== matlab function MPC/3 - Navigation/Subsystem/STDQMEKF/MATLAB Function3 ==
  data: u input; x output
function x = fcn(u)
dq = [u(1:4),u(5:8)];
dv = [[0; u(9:11)], [0; u(12:14)]];
if norm(dq(:,1)) == 0
    dq = zeros(4,2);
    dq(1,1) = 1;
end
[q,r] = dq2quat(dq,'scalarFirst');
q = smallQuat(q,'scalarFirst');
v = dqLinearVelocity(dv, dq);
w = dv(2:4,1);
x = [q; r'; -w; -v];
end

function v_world = dqLinearVelocity(dq_vel, dq_pose)


    %-- 1) body‐frame linear velocity (pure quaternion) --%
    % Conjugate of the pose rotation quaternion:
    q_r_conj = quatConj(dq_pose(:,1),'scalarFirst');
    
    % pure‐quat v_body_q = 2 * (qv_dual * conj(q_pose.r))
    v_body_quat = 2 * quatMultiply(dq_vel(:,2), q_r_conj,'scalarFirst');
    
    %-- 2) rotate into world frame --%
    % dqRotate(q, p) ≡ q * p * conj(q) v_body_quat(2:4)
    v_world_quat = quatRotate(dq_pose(:,1), v_body_quat(2:4),'scalarFirst');
    
    %-- 3) extract vector part --%
    v_world = v_world_quat;

end

== matlab function MPC/4 - Control/Default PD Control (RED)/Homo/MATLAB Function4 ==
  data: q1 input; u output; k1t parameter; alphat parameter
function u = fcn(q1,k1t, alphat)

u = k1t*sign(q1)*(abs(q1)^(alphat/(2 - alphat)));

== matlab function MPC/3 - Navigation/Subsystem/STQMEKF/MATLAB Function1 ==
  data: dt input; RED_quat input; RED_x input; BLACK_q input; BLACK_x input; x_est output; x_prev input; P_prev input; P_est output; compT output; y output; NIS output; V_prev input; V_est output; Q parameter; R parameter; maxd parameter; rho parameter
function [x_est, P_est, compT, y, NIS, V_est] = QMEKF(dt, RED_quat, RED_x, BLACK_q, BLACK_x, x_prev, P_prev, V_prev, Q, R, maxd, rho)

%% Best QMEKF values
s1 = 1e-6;
s2 = 1e-6;
s3 = 1e-10;
s4 = 1e-7 ;
s5 = 0.06;
s6 = 0.001 ;
s7 = s6;

d1 = 1.6046;
d2 = 5.5866;
rho = 0.98;

Q = blkdiag(s1*eye(3), s2*eye(3), s3*eye(3), s4*eye(3));


R = blkdiag(s5*eye(3), s6, s7*eye(2));

maxd = [d1
        d2];

%%
r = 0;
z = [BLACK_q; BLACK_x];
Chaser = [RED_quat; RED_x];

tic
[y, H, x_est, P_est, V_est] = runSTQMEKF(z, dt, Chaser, ...
       x_prev, P_prev, V_prev, Q, R, r, rho, maxd);
compT = toc;

% Assume H is the full measurement matrix
S_att = H * P_est * H' + R;
NIS = y' / S_att * y;
end

== matlab function MPC/3 - Navigation/Subsystem/STQMEKF/MATLAB Function2 ==
  data: u input; out output
function out = fcn(u)

y = u;

y(1:4) = smallQuat(u(1:4),'scalarFirst');
y(5:7) = -1*u(5:7);

out = [y(1:4); y(8:10); y(5:7); y(11:13)];

== matlab function MPC/3 - Navigation/Subsystem/STRMEKF/MATLAB Function ==
  data: x input; out output; q input
function out = fcn(x,q)

y = [q;x];
y(1:4) = smallQuat(y(1:4),'scalarFirst');

out = [y(1:7); y(11:13); y(8:10)];

== matlab function MPC/Simulate Plant Dynamics/RED and ARM Dynamics/RED Only/Calculated & Store Measured States/Subsystem2/Enabled Subsystem/MATLAB Function ==
  data: y input; dy output; dt input; tau input; dy_prev input; ema_prev input; ema output
function [dy, ema] = realtime_derivative_ema(y, dt, tau, dy_prev, ema_prev)
    % Inputs:
    % y: Current measurement
    % dt: Time step
    % alpha: Smoothing factor (e.g., 0.1)

    alpha = 1 - exp(-dt / tau);
        
    % Update EMA
    ema = alpha.*y + (1 - alpha).*ema_prev;
    
    % Compute derivative
    dy = (ema - ema_prev)./dt;
    
end

== matlab function MPC/3 - Navigation/Subsystem/STRMEKF/MATLAB Function1 ==
  data: dt input; RED_yaw input; RED_x input; VIS_R input; VIS_x input; x_est output; Rot_est output; x_prev input; Rot_prev input; P_prev input; P_est output; compT output; y output; NIS output; V_est output; V_prev input; Q parameter; R parameter; maxd parameter
function [x_est, Rot_est, P_est, compT, y, NIS, V_est] = RMEKF(dt, RED_yaw, RED_x, VIS_R, VIS_x, x_prev, Rot_prev, P_prev, V_prev, Q, R, maxd)

s1 = 1e-2; % quat
s2 = 1e-4; % angular vel
s3 = 1e-10; % position
s4 = 1e-7; % velocity
s5 = 0.006; % quat meas 
s6 = 0.001 ; % position meas
s7 = s6; 

d1 = 1.6046;
d2 = 5.5866;
rho = 0.98;

Q = blkdiag(s1*eye(3), s3*eye(3), s4*eye(3), s2*eye(3));


R = blkdiag(s5*eye(3), s6, s7*eye(2));

maxd = 1000*[d1
        d2];

rho = 0.98;

r = 0;
z = VIS_x;
Chaser = [RED_x(1:2); RED_yaw];

tic
[x_est, Rot_est, P_est, y, H, V_est] = runSTRMEKF(Chaser, z, VIS_R, dt, x_prev, Rot_prev, P_prev, Q, R, V_prev, r, rho, maxd);

compT = toc;

% Calc NIS
Pzz = H*P_est*H' + R;
NIS = y' / Pzz * y;

end

== matlab function MPC/3 - Navigation/Subsystem/STRMEKF/MATLAB Function11 ==
  data: u input; y output
function y = fcn(u)
if det(u) == 0
    u = eye(3);
end
u(1:2,1:2) = u(1:2,1:2);
y = rotm2Quat(u','scalarFirst');

== matlab function MPC/3 - Navigation/Subsystem/Filter Error/MATLAB Function ==
  data: true input; y output; est input
function y = fcn(true, est)
true(1:4) = normalizeQuat(true(1:4),'scalarFirst');
q = quatInv(true(1:4),'scalarFirst');
q = quatMultiply(q,est(1:4),'scalarFirst');
q = smallQuat(q,'scalarFirst');
mrp = quat2mrp(q,1,1,'scalarFirst');

temp = true(5:end) - est(5:end);

y = [mrp(3); temp(1:2); temp(6); temp(7:8)];

== matlab function MPC/3 - Navigation/Subsystem/Filter Error/MATLAB Function1 ==
  data: true input; y output; est input
function y = fcn(true, est)
true(1:4) = normalizeQuat(true(1:4),'scalarFirst');
q = quatInv(true(1:4),'scalarFirst');
q = quatMultiply(q,est(1:4),'scalarFirst');
q = smallQuat(q,'scalarFirst');
mrp = quat2mrp(q,1,1,'scalarFirst');

temp = true(5:end) - est(5:end);

y = [mrp(3); temp(1:2); temp(6); temp(7:8)];

== matlab function MPC/4 - Control/Default PD Control (RED)/Homo/MATLAB Function5 ==
  data: q2 input; u output; k2t parameter; alphat parameter
function u = fcn(q2,k2t, alphat)

u = k2t*sign(q2)*(abs(q2)^alphat);

== matlab function MPC/4 - Control/Default PD Control (RED)/LQR/MATLAB Function ==
  data: k input; u output; q1_x input; q2_x input; q1_y input; q2_y input; q1_t input; q2_t input
function u = fcn(k,q1_x,q2_x,q1_y,q2_y,q1_t,q2_t)

x = [q1_x;
    q1_y;
    q1_t;
    q2_x;
    q2_y;
    q2_t];

u = k*x;
% u = [0; 0; 0];

== matlab function MPC/4 - Control/Default PD Control (RED)/Min Energy/MATLAB Function ==
  data: q1 input; u output; q2 input; Tf parameter; m parameter; t input; dt output
function [u,dt] = fcn(q1,q2,Tf, m,t)
dt = Tf-t;
if t < Tf
    u1 = -6*m*q1/((Tf-t)^2);
    u2 = -4*m*q2/(Tf-t);
    
    u = u1 + u2;
    u = -1*u;
else
    u = 0;
end

== matlab function MPC/4 - Control/Default PD Control (RED)/Min Energy/MATLAB Function1 ==
  data: q1 input; u output; q2 input; Tf parameter; m parameter; t input; dt output
function [u,dt] = fcn(q1,q2,Tf, m,t)
dt = Tf-t;
if t < Tf
    u1 = -6*m*q1/((Tf-t)^2);
    u2 = -4*m*q2/(Tf-t);
    
    u = u1 + u2;
    u = -1*u;
else
    u = 0;
end

== matlab function MPC/4 - Control/Default PD Control (RED)/Min Energy/MATLAB Function2 ==
  data: q1 input; u output; q2 input; Tf parameter; J parameter; t input; dt output
function [u,dt] = fcn(q1,q2,Tf, J,t)
dt = Tf - t;
if t < Tf
    u1 = -6*J*q1/((Tf-t)^2);
    u2 = -4*J*q2/(Tf-t);
    
    u = u1 + u2;
    u = -1*u;
else
    u = 0;
end

== matlab function MPC/4 - Control/Default PD Control (RED)/Minimum Time Controller/MATLAB Function ==
  data: q_1 input; sign_Argument output; q_2 input; F_max parameter; M parameter
function sign_Argument = fcn(q_1, q_2, F_max, M)

sign_Argument = q_2 + sign(q_1) * sqrt(2 * abs(q_1) * F_max / M);

== matlab function MPC/4 - Control/Default PD Control (RED)/Minimum Time Controller/MATLAB Function1 ==
  data: q_1 input; sign_Argument output; q_2 input; F_max parameter; M parameter
function sign_Argument = fcn(q_1, q_2, F_max, M)

sign_Argument = q_2 + sign(q_1) * sqrt(2 * abs(q_1) * F_max / M);

== matlab function MPC/Simulate Plant Dynamics/BLACK Dynamics/Calculated & Store Measured States/Subsystem1/Enabled Subsystem/MATLAB Function ==
  data: y input; dy output; dt input; tau input; dy_prev input; ema_prev input; ema output
function [dy, ema] = realtime_derivative_ema(y, dt, tau, dy_prev, ema_prev)
    % Inputs:
    % y: Current measurement
    % dt: Time step
    % alpha: Smoothing factor (e.g., 0.1)

    alpha = 1 - exp(-dt / tau);
        
    % Update EMA
    ema = alpha.*y + (1 - alpha).*ema_prev;
    
    % Compute derivative
    dy = (ema - ema_prev)./dt;
    
end

== matlab function MPC/4 - Control/Default PD Control (RED)/Minimum Time Controller/MATLAB Function2 ==
  data: q_1 input; sign_Argument output; q_2 input; T_max parameter; J parameter
function sign_Argument = fcn(q_1, q_2, T_max, J)

sign_Argument = q_2 + sign(q_1) * sqrt(2 * abs(q_1) * T_max / J);

== matlab function MPC/4 - Control/Default PD Control (RED)/Minimum Time Controller/MATLAB Function3 ==
  data: q_1 input; sign_Argument input; u_max_product output
function u_max_product = fcn(q_1, sign_Argument)

if sign_Argument == 0

    u_max_product = sign(q_1);

else

    u_max_product = sign(sign_Argument);

end

== matlab function MPC/4 - Control/Default PD Control (RED)/Minimum Time Controller/MATLAB Function4 ==
  data: q_1 input; sign_Argument input; u_max_product output
function u_max_product = fcn(q_1, sign_Argument)

if sign_Argument == 0

    u_max_product = sign(q_1);

else

    u_max_product = sign(sign_Argument);

end

== matlab function MPC/4 - Control/Default PD Control (RED)/Minimum Time Controller/MATLAB Function5 ==
  data: q_1 input; sign_Argument input; u_max_product output
function u_max_product = fcn(q_1, sign_Argument)

if sign_Argument == 0

    u_max_product = sign(q_1);

else

    u_max_product = sign(sign_Argument);

end

== matlab function MPC/4 - Control/Default PD Control (RED)/SAC/Diff/Hough Control/MATLAB Function2 ==
  data: Oy output; z input; Ox output
function [Oy, Ox]   = C3( z )
%C3 gives the rotation matrix about the z-axis for an angle 'z'
%   z - the angle about the z-axis which you rotate
%   A - the rotation matrix

Ox = [cos(z) sin(z); -sin(z) cos(z)]*[1;0];
Oy = [cos(z) sin(z); -sin(z) cos(z)]*[0;1];
end

== matlab function MPC/4 - Control/Default PD Control (RED)/SAC/Diff/Hough Control/MATLAB Function3 ==
  data: z input; Ox output
function Ox    = C3( z )
%C3 gives the rotation matrix about the z-axis for an angle 'z'
%   z - the angle about the z-axis which you rotate
%   A - the rotation matrix

Ox = [cos(z) sin(z); -sin(z) cos(z)]*[1;0];
end

== matlab function MPC/4 - Control/Default PD Control (RED)/SAC/Diff/Hough Control/MATLAB Function4 ==
  data: Oy input; e_out output; e_in input
function e_out = fcn(Oy, e_in)

a = sign(Oy'*e_in);
e_out = -a*norm(e_in);

== matlab function MPC/4 - Control/Default PD Control (RED)/SAC/Ideal Plant Model2/MATLAB Function ==
  data: u input; y output
function y = fcn(u)

y = u(1);

== matlab function MPC/4 - Control/Default PD Control (RED)/SAC/Ideal Plant Model2/MATLAB Function1 ==
  data: u input; y output
function y = fcn(u)

y = u(1);

== matlab function MPC/4 - Control/Default PD Control (RED)/SAC/SAC_CTL/Position/Storage/MATLAB Function3 ==
  data: u input; y1 output; y2 output; y3 output; y4 output
function [y1,y2,y3,y4] = fcn(u)
y1 = u(1);
y2 = u(2);
y3 = u(3);
y4 = u(4);
end

== matlab function MPC/4 - Control/Default PD Control (RED)/SAC/SAC_CTL/Angle/MATLAB Function ==
  data: um input; u output; xm input; ey input; Ke_l input size=1; Kx_l input; Ku_l input; Ke output size=1; Kx output size=1,2; Ku output; Kedot_l output; Kxdot_l output; Kudot_l output; gamma_I_t parameter; gamma_P_t parameter; sigma_sac_t parameter
function [u, Ke, Kx, Ku, Kedot_l, Kxdot_l, Kudot_l] = sac(um, xm, ey, Ke_l, Kx_l, Ku_l,gamma_I_t, gamma_P_t, sigma_sac_t)
% gamma_I = [451300 0 0; 0 0 0; 0 0 0] ;
% gamma_P = 3.5*[122500 0 0; 0 534500 0; 0 0 258000] ;
% sigma_sac = 0.93 ;

%%% Ke
Kpe = ey*ey'*gamma_P_t(1,1) ;
Kedot_l = ey*ey'*gamma_I_t(1,1) - sigma_sac_t*Ke_l ;
Ke = Kpe + Ke_l ;

%%% Kx
Kpx = ey*xm'*gamma_P_t(2,2) ;
Kxdot_l = ey*xm'*gamma_I_t(2,2) ;
Kx = Kpx + Kx_l ;

%%% Ku
Kpu = ey*um'*gamma_P_t(3,3) ;
Kudot_l = ey*um'*gamma_I_t(3,3) ;
Ku = Kpu + Ku_l ;

%%% input
u = Ke*ey + Kx*xm + Ku*um ;
end

== matlab function MPC/4 - Control/Default PD Control (RED)/SAC/SAC_CTL/MATLAB Function ==
  data: um input; ump output; xm input; ey input; xmp output; eyp output; umt output; xmt output; eyt output
function [ump,xmp,eyp,umt,xmt,eyt] = fcn(um,xm,ey)
ump = um(1:2);
umt = um(3);
xmp = xm([1:2,4:5]);
xmt = xm([3,6]);
eyp = ey(1:2);
eyt = ey(3);
end

== matlab function MPC/Simulate Plant Dynamics/RED and ARM Dynamics/RED Only/Data @ Measurement Rate/Calculate True Time Step/MATLAB Function ==
  data: dt input; dt_out output; dataRate input
function dt_out = CheckforInvalidTime(dt, dataRate)

    if dt <= 0

        dt_out = dataRate;

    else

        dt_out = dt;

    end


end

== matlab function MPC/4 - Control/Default PD Control (RED)/SAC/SAC_CTL/Position/MATLAB Function1 ==
  data: um input; u output; xm input; ey input; Ke_l input; Kx_l input; Ku_l input; Ke output size=2,2; Kx output size=2,4; Ku output size=2,2; Kedot_l output; Kxdot_l output; Kudot_l output; gamma_I parameter; gamma_P parameter; sigma_sac parameter
function [u, Ke, Kx, Ku, Kedot_l, Kxdot_l, Kudot_l] = sac(um, xm, ey, Ke_l, Kx_l, Ku_l,gamma_I, gamma_P, sigma_sac)
% gamma_I = [451300 0 0; 0 0 0; 0 0 0] ;
% gamma_P = 3.5*[122500 0 0; 0 534500 0; 0 0 258000] ;
% sigma_sac = 0.93 ;

%%% Ke
Kpe = ey*ey'*gamma_P(1,1) ;
Kedot_l = ey*ey'*gamma_I(1,1) - sigma_sac*Ke_l ;
Ke = Kpe + Ke_l ;

%%% Kx
Kpx = ey*xm'*gamma_P(2,2) ;
Kxdot_l = ey*xm'*gamma_I(2,2) ;
Kx = Kpx + Kx_l ;

%%% Ku
Kpu = ey*um'*gamma_P(3,3) ;
Kudot_l = ey*um'*gamma_I(3,3) ;
Ku = Kpu + Ku_l ;

%%% input
u = Ke*ey + Kx*xm + Ku*um ;
end

== matlab function MPC/4 - Control/Default PD Control (RED)/SMC/MATLAB Function ==
  data: e input; u output; de input; k_p parameter; lambda_p parameter; m parameter
function u = fcn(e,de,k_p, lambda_p,m)
u = lambda_p*m*de + k_p*custom_sign(lambda_p*m*de + e*m);
end

function s = custom_sign(x)
    % custom_sign returns the sign of each element in the input array x.
    % Output s has the same dimensions as x, where:
    % s(i) is -1 if x(i) < 0
    % s(i) is  1 if x(i) > 0
    % s(i) is  0 if x(i) == 0
    
    % Preallocate the output array
    s = zeros(size(x));
    
    % Set elements to -1 where x is less than 0
    s(x < 0) = -1;
    
    % Set elements to 1 where x is greater than 0
    s(x > 0) = 1;
end

== matlab function MPC/4 - Control/Default PD Control (RED)/SMC/MATLAB Function1 ==
  data: e input; u output; de input; k_p parameter; lambda_p parameter; m parameter
function u = fcn(e,de,k_p, lambda_p,m)
u = lambda_p*m*de + k_p*sign(lambda_p*m*de + e*m);
end

== matlab function MPC/4 - Control/Default PD Control (RED)/SMC/MATLAB Function2 ==
  data: e input; u output; de input; k_t parameter; lambda_t parameter; J parameter
function u = fcn(e,de,k_t, lambda_t,J)
u = lambda_t*J*de + k_t*sign(lambda_t*J*de + J*e);
end

== matlab function MPC/4 - Control/Default PD Control (RED)/Sat/MATLAB Function ==
  data: q2 input; q1 input; saturation output; a1 parameter; b parameter; m parameter
function saturation = fcn(q2,q1,a1, b, m)

u = a1*m*q1 + a1*m*q2/b;

saturation = u;

== matlab function MPC/4 - Control/Default PD Control (RED)/Sat/MATLAB Function1 ==
  data: q2 input; q1 input; saturation output; a1 parameter; b parameter; m parameter
function saturation = fcn(q2,q1,a1, b, m)

u = a1*m*q1 + a1*m*q2/b;

saturation = u;

== matlab function MPC/4 - Control/Default PD Control (RED)/Sat/MATLAB Function2 ==
  data: q2 input; q1 input; saturation output; c parameter; d parameter; J parameter
function saturation = fcn(q2,q1,c, d, J)

u = c*J*q1 + c*J*q2/d;

saturation = u;

== matlab function MPC/Model Predictive Control/Model Predictive Control/Compute P matrix, and h vector (ALL Inequality Constraints) ==
  data: F_h input; f_h input; F_c input; f_c input; F_v parameter; f_v input; F_u parameter; f_u parameter; P output; h output; F_t parameter; f_t parameter; use_table_constr parameter; use_LOS_constr parameter
function [P, h] = fcn(F_h, f_h, F_c, f_c, F_v, f_v, F_u, f_u, F_t, f_t, use_table_constr, use_LOS_constr)

if ~use_table_constr
    F_t = zeros(size(F_t));
    f_t = zeros(size(f_t));
end

if ~use_LOS_constr
    F_v = zeros(size(F_v));
    f_v = zeros(size(f_v));
end

P = [F_u; F_h; F_c; F_t; F_v];
h = [f_u; f_h; f_c; f_t; f_v];

end

== matlab function MPC/4 - Control/Default PD Control (RED)/Sat/MATLAB Function3 ==
  data: q2 input; u input; saturation output; F_max parameter; e parameter; b parameter; m parameter
function saturation = fcn(q2,u,F_max, e, b, m)

if u >= e
    u = e;
elseif u <= -1*e
    u = -1*e;
else
    u = u;
end

u = b*q2*m + u;

if u >= F_max
    u = F_max;
elseif u <= -1*F_max
    u = -1*F_max;
else
    u = u;
end

saturation = u;

== matlab function MPC/4 - Control/Default PD Control (RED)/Sat/MATLAB Function4 ==
  data: q2 input; u input; saturation output; F_max parameter; b parameter; m parameter; e parameter
function saturation = fcn(q2,u,F_max, b, m, e)

if u >= e
    u = e;
elseif u <= -1*e
    u = -1*e;
else
    u = u;
end

u = b*q2*m + u;

if u >= F_max
    u = F_max;
elseif u <= -1*F_max
    u = -1*F_max;
else
    u = u;
end

saturation = u;
